simulink model "Simul_Controlador"  (R2020b)
settings: Solver=VariableStepAuto  StartTime=0.0  StopTime=10.0  RelTol=1e-3
values from neighbouring files (symbols this model uses):
  h = 0.05    [Unity3Dsimulacion.m]
  X0 = [0 0.5 0 0 0]    [Unity3Dsimulacion.m]
libraries: cstblocks x1
settings Model: Creator=Eduard  LastModifiedBy=Eduard

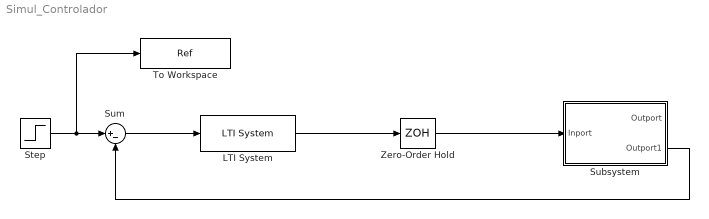
== system Simul_Controlador ==
  LTI System : cstblocks/LTI System  sys=Controller  IC=[]
  Step : Step  Time=0  After=0.5  SampleTime=0
  Subsystem : Subsystem
  Sum : Sum  Inputs=|+-
  To Workspace : ToWorkspace  VariableName=Ref  SaveFormat=Structure With Time  SampleTime=h
  Zero-Order Hold : ZeroOrderHold  SampleTime=h
  wires:
  Step/1 -> To Workspace/1, Sum/1
  Sum/1 -> LTI System/1
  LTI System/1 -> Zero-Order Hold/1
  Zero-Order Hold/1 -> Subsystem/1(Inport)
  Subsystem/2(Outport1) -> Sum/2

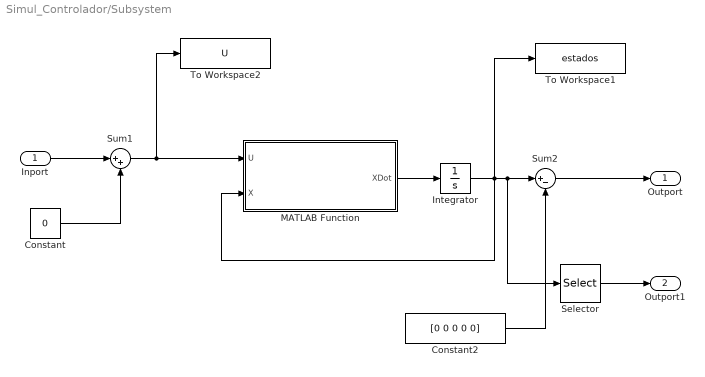
== system Simul_Controlador/Subsystem ==
  Inport : Inport
  Constant : Constant  Value=0
  Constant2 : Constant  Value=[0 0 0 0 0]
  Integrator : Integrator  InitialCondition=X0
  MATLAB Function : MATLAB Function  TreatAsAtomicUnit=on
  Selector : Selector  InputPortWidth=5  IndexOptions=Index vector (dialog)  Indices=2  OutputSizes=1
  Sum1 : Sum  Inputs=|++
  Sum2 : Sum  Inputs=|+-
  To Workspace1 : ToWorkspace  VariableName=estados  SaveFormat=Structure With Time  SampleTime=h
  To Workspace2 : ToWorkspace  VariableName=U  SaveFormat=Structure With Time  SampleTime=h
  Outport : Outport
  Outport1 : Outport  Port=2
  wires:
  Integrator/1 -> To Workspace1/1, MATLAB Function/2(X), Selector/1, Sum2/1
  Constant/1 -> Sum1/2
  MATLAB Function/1(XDot) -> Integrator/1
  Sum1/1 -> To Workspace2/1, MATLAB Function/1(U)
  Inport/1 -> Sum1/1
  Sum2/1 -> Outport/1
  Constant2/1 -> Sum2/2
  Selector/1 -> Outport1/1

== matlab function Simul_Controlador/Subsystem/MATLAB Function ==
  data: U input; XDot output; X input
function XDot = ball_and_beam_model(U,X)
%#codegen
% Constants of the model
[m,J,r,g]           = deal(0.1,0.025,0.01,9.807);

%% State space model
% x1 = theta, x2  = x, x3 = thetadot, x4 = xdot
[X1,X2,X3,X4]= deal(X(1),X(2),X(3),X(4));

% Inertia matrix
D           = [m*r^2+m*X2^2+J, -m*r; -m*r, m];

% Coriolis and centrifugal forces
H           = [2*m*X2*X4*X3; -m*X2*X3^2];

% Gravity forces
G           = [m*g*X2*cos(X1)-m*g*r*sin(X1); m*g*sin(X1)];

% Generalized effort
E           = [U; 0];

% Derivatives of states
XDot        = [X3; X4; D\(E-H-G)];
end
